simulink model "HeliModel"  (R2022b)
settings: Solver=VariableStepAuto  StartTime=0.0  StopTime=10.0  RelTol=1e-3
settings Model: Creator=henrr  LastModifiedBy=henrr

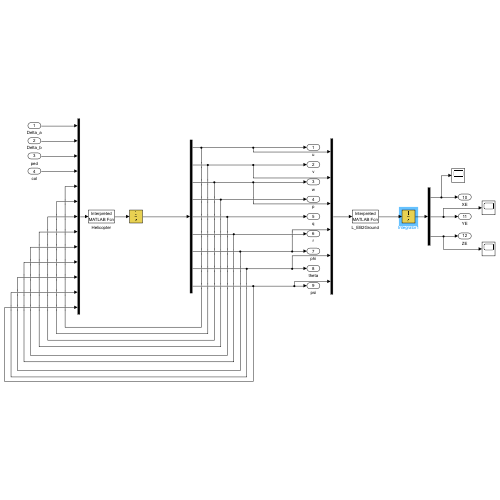
[thumbnail: Simulink's stored preview of the top-level diagram]
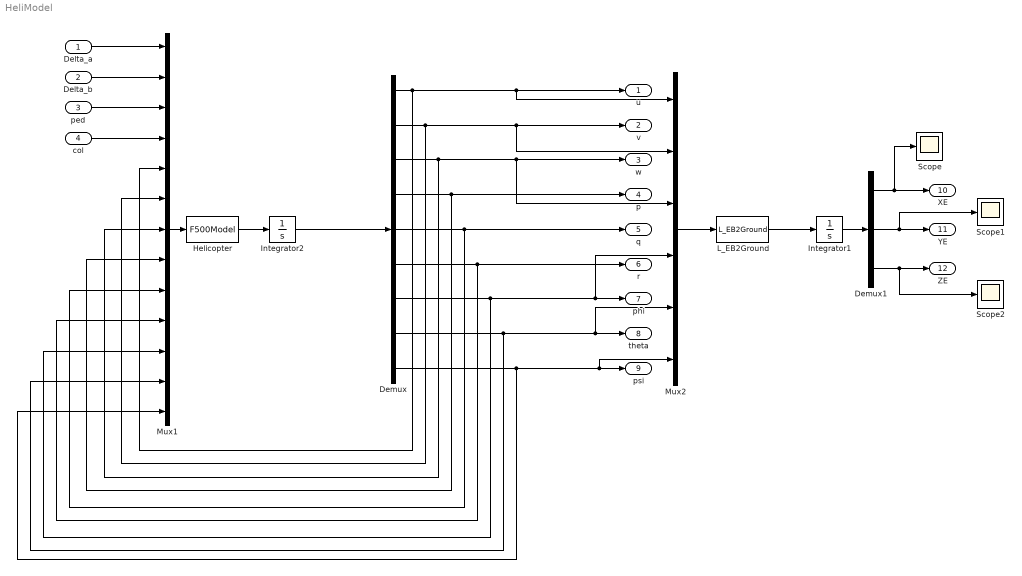
== system HeliModel ==
  Delta_a : Inport
  Delta_b : Inport  Port=2
  ped : Inport  Port=3
  col : Inport  Port=4
  Demux : Demux  Outputs=9
  Demux1 : Demux  Outputs=3
  Helicopter : MATLABFcn  MATLABFcn=F500Model
  Integrator1 : Integrator  InitialCondition=[0 0 0]
  Integrator2 : Integrator  InitialCondition=[0 0 0 0 0 0 0 0 0]
  L_EB2Ground : MATLABFcn  MATLABFcn=L_EB2Ground
  Mux1 : Mux  Inputs=13
  Mux2 : Mux  Inputs=6
  Scope : Scope
  Scope1 : Scope
  Scope2 : Scope
  u : Outport
  v : Outport  Port=2
  w : Outport  Port=3
  p : Outport  Port=4
  q : Outport  Port=5
  r : Outport  Port=6
  phi : Outport  Port=7
  theta : Outport  Port=8
  psi : Outport  Port=9
  XE : Outport  Port=10
  YE : Outport  Port=11
  ZE : Outport  Port=12
  wires:
  Demux/9 -> Mux1/13, psi/1, Mux2/6
  Delta_b/1 -> Mux1/2
  Demux/5 -> Mux1/9, q/1
  Mux1/1 -> Helicopter/1
  ped/1 -> Mux1/3
  Demux/8 -> Mux1/12, theta/1, Mux2/5
  Demux/1 -> Mux1/5, u/1, Mux2/1
  Helicopter/1 -> Integrator2/1
  Integrator2/1 -> Demux/1
  Demux/7 -> Mux1/11, phi/1, Mux2/4
  Mux2/1 -> L_EB2Ground/1
  Integrator1/1 -> Demux1/1
  Demux/4 -> Mux1/8, p/1
  Demux/6 -> Mux1/10, r/1
  Demux1/1 -> XE/1, Scope/1
  Demux/2 -> Mux1/6, v/1, Mux2/2
  col/1 -> Mux1/4
  Demux1/2 -> YE/1, Scope1/1
  Demux/3 -> Mux1/7, w/1, Mux2/3
  L_EB2Ground/1 -> Integrator1/1
  Delta_a/1 -> Mux1/1
  Demux1/3 -> ZE/1, Scope2/1
